simulink model "tqdtqr_rebuild_V3"  (R2021b)
settings: Solver=VariableStepAuto  StartTime=0.0  StopTime=10.0  RelTol=1e-3
undefined symbols (not defined in the file): ATQD_AfterTqMinGain_X_Deg, ATQD_APSCreepBaseTqD_X_kph, ATQD_APSCreepBaseTqD_Y_Deg, ATQD_APSCreepBaseTqR_X_kph, ATQD_APSCreepBaseTqR_Y_Deg, ATQD_APSCreepIterm_X_kph, ATQD_APSCreepIterm_Y_kph, ATQD_APSCreepPterm_X_kph, ATQD_APSCreepPterm_Y_kph, ATQD_APSDecReq_X_kph, ATQD_APSDecReq_Y_mps2, ATQD_APSDecReqCMD_X_kph, ATQD_APSDecReqTs_X_pct, ATQD_APSDecTimeGain_X_Deg, ATQD_APSDecTimeGain_Y_s, ATQD_APSReqLowSpd_X_Deg, ATQD_AutoHoldReleaseBPS_X_Deg, ATQD_AWDLoadTrqnsGain_X_kg, ATQD_AWDLoadTrqnsGain_Y_pct, ATQD_BOSEnBPSPosn_X_kph, ATQD_BOSMap_X_rpm, ATQD_BOSMap_Y_pct, ATQD_CreepBaseTqD_X_kph, ATQD_CreepBaseTqD_Y_Deg, ATQD_CreepBaseTqR_X_kph, ATQD_CreepBaseTqR_Y_Deg, ATQD_CreepBPSDisPosn_X_Deg, ATQD_CreepBPSDisPosnR_X_Deg, ATQD_CreepBPSEnPosn_X_Deg, ATQD_CreepBPSEnPosnR_X_Deg, ATQD_CreepDeltaTq_X_kph, ATQD_CreepIterm_X_kph, ATQD_CreepIterm_Y_kph, ATQD_CreepItermMaxLimit_X_pct, ATQD_CreepPreloadTime_X_kph, ATQD_CreepPreloadTq_X_kph, ATQD_CreepPreloadTq_Y_s, ATQD_CreepProtTq_X_Deg, ATQD_CreepPterm_X_kph, ATQD_CreepPterm_Y_kph, ATQD_CreepRrTqSpRat_X_rpm, ATQD_CreepRrTqSpRat_Y_Nm, ATQD_CreepTargetSpdD_X_pct, ATQD_CreepTargetSpdR_X_pct, ATQD_CreepUpLimitTq_X_rpm, ATQD_DecIneOPDHoldEnDelay_X_Deg, ATQD_DecIneOPDHoldEnDelay_Y_bar, ATQD_ECOTqMapD_X_rpm, ATQD_ECOTqMapD_Y_pct, ATQD_EMTqMapD_X_rpm, ATQD_EMTqMapD_Y_pct, ATQD_EOPDTqMapDCon_X_rpm, ATQD_EOPDTqMapDCon_Y_Deg, ATQD_EstInitVehWeight_X_c, ATQD_FAfterTqCMDGain_X_rpm, ATQD_FAfterTqCMDGain_Y_pct, ATQD_ForceLowSpd_X_Deg, ATQD_ForcePLimitSpd_X_Deg, ATQD_FrLossMAPLowV_X_rpm, ATQD_FrLossMAPLowV_Y_Nm ... (+949)
libraries: simulink x235, hcu_lib x208, tqr x63, tqd x6
(part 14 of 37)

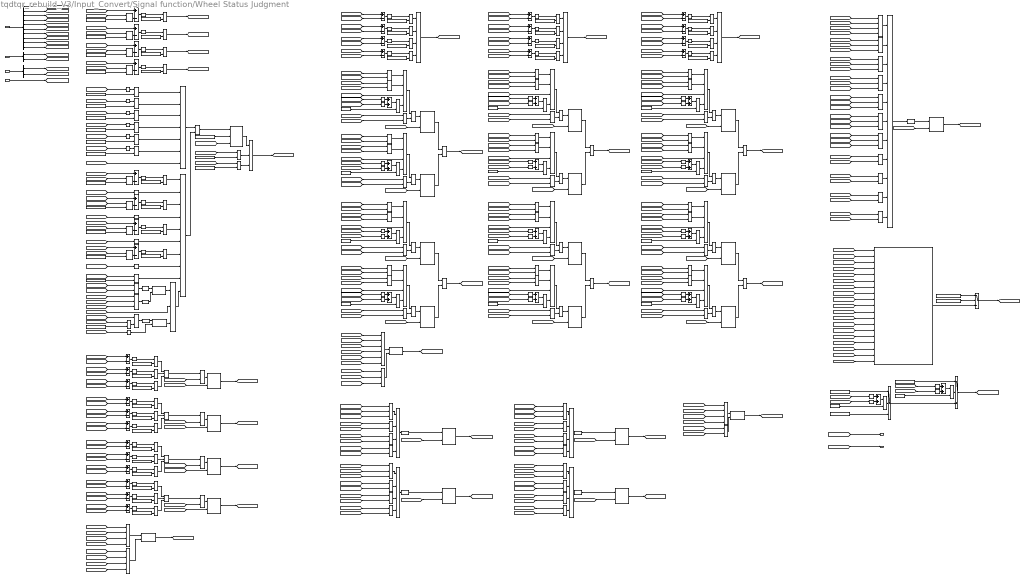
== system tqdtqr_rebuild_V3/Input_Convert/Signal function/Wheel Status Judgment ==
  note: Each wheel speed getting bigger and bigger
  note: Stable Reset Judgment
  note: Double wheels skip
  note: Skip Direction
  note: Single wheel skip
  note: Find out which wheels skip
  note: Tripple wheels skip
  note: All wheels skip
  BSCPIn_outputs : Inport
  BSignalConvert_outputs : Inport  Port=2
  BMain_outputs : Inport  Port=3
  VTQD_GearActualPosn_enum : Inport  Port=4
  AND : Logic  Inputs=7  AllPortsSameDT=off  OutDataTypeStr=boolean
  AND1 : Logic  Inputs=10  AllPortsSameDT=off  OutDataTypeStr=boolean
  AND{8,10..12,14,17,19,21,23,26,28,30,32,35..37,39..41,43..45,47..49,57..60} (29 alike) : Logic  AllPortsSameDT=off  OutDataTypeStr=boolean
  AND{6..7,9,13,15..16,18,20,22,24..25,27,29,31,33,50} (16 alike) : Logic  Inputs=4  AllPortsSameDT=off  OutDataTypeStr=boolean
  AND{2..5,34,38,42,46,51..56} (14 alike) : Logic  Inputs=3  AllPortsSameDT=off  OutDataTypeStr=boolean
  Abs{,1..37} (38 alike) : Abs
  Add{,1..23,28..31,36..39} (32 alike) : Sum  Inputs=+-
  Add{24..27,32..35,40..45} (14 alike) : Sum
  Bus Selector : BusSelector  OutputSignals=task_time_s,VINP_LFRawWhlSpeed_kph,VINP_LRRawWhlSpeed_kph,VINP_RFRawWhlSpeed_kph,VINP_RRRawWhlSpeed_kph,VINP_VehSpeed_kph,VINP_FrPTCSActive_flg,VINP_RrPTCSActive_flg,VTQD_LowIdleAccPedal_flg,VINP_DIDGetDynoMode_flg
  Bus Selector1 : BusSelector  OutputSignals=VTQD_BrkSwSta_flg,VTQD_VehActSpd_kph
  Bus Selector2 : BusSelector  OutputSignals=VTQR_NoABSFEDUWhlTqReq_Nm,VTQR_NoABSREDUWhlTqReq_Nm
  Constant{1..6,16} (7 alike) : Constant  Value=KTQD_WhlEnDetStableSpd_kph
  Constant{8,10,12,14,30,32,34,71} (8 alike) : Constant  Value=KTQD_RocModeWhlSpdDely_cnt
  Constant{9,11,13,15,17..29,38..40,46..49,54..57} (28 alike) : Constant  Value=KTQD_WhlSpeedStableDev_kph
  Constant{31,33,35..36} (4 alike) : Constant  Value=KTQD_RocModeTqLimSpdDev_kph
  Constant{41..42,44..45,50..53,58..61,64..65} (14 alike) : Constant  Value=ZERO_FLOAT
  Constant43 : Constant  Value=KTQD_FreeWhlDetStableSpd_kph
  Constant62 : Constant  Value=ENUM_GEARACTUALPOSN_N
  Constant63 : Constant  Value=ENUM_GEARACTUALPOSN_P
  Constant66 : Constant  Value=ENUM_SKIPDIRECT_NONE
  Constant67 : Constant  Value=ENUM_SKIPDIRECT_NEGATIVE
  Constant68 : Constant  Value=ENUM_SKIPDIRECT_POSITIVE
  Constant69 : Constant  Value=KTQD_ActWhlSkipSta_enum_ovrdflg
  Constant7 : Constant  Value=KTQD_WhlStableDetTime_s
  Constant70 : Constant  Value=KTQD_ActWhlSkipSta_enum_ovrdval
  Delay{,9..35} (28 alike) : Delay  DelayLength=1  InitialCondition=single(0.0)
      settings: AttributesFormatString=%<InitialCondition>
  Delay{1..8} (8 alike) : Delay  DelayLengthSource=Input port
      settings: InputPortMap=u0,p1
  DelayEnable : hcu_lib/Basic_Blocks/DelayEnable
  Detect Decrease : simulink/Logic and Bit Operations/Detect Decrease  vinit=boolean(0)  OutDataTypeStr=boolean
  Detect Increase{,1..6} (7 alike) : simulink/Logic and Bit Operations/Detect Increase  vinit=boolean(0)  OutDataTypeStr=boolean
  Equal : RelationalOperator  Operator===  OutDataTypeStr=boolean  RndMeth=Simplest
  Equal1 : RelationalOperator  Operator===  OutDataTypeStr=boolean  RndMeth=Simplest
  NOT{,1..4} (5 alike) : Logic  Operator=NOT  AllPortsSameDT=off  OutDataTypeStr=boolean
  OR{,1..4,7..10,13..21,24..29,36} (25 alike) : Logic  Operator=OR  AllPortsSameDT=off  OutDataTypeStr=boolean
  OR{11..12,23,30} (4 alike) : Logic  Operator=OR  Inputs=3  AllPortsSameDT=off  OutDataTypeStr=boolean
  OR22 : Logic  Operator=OR  Inputs=6  AllPortsSameDT=off  OutDataTypeStr=boolean
  OR{5..6,31..35} (7 alike) : Logic  Operator=OR  Inputs=4  AllPortsSameDT=off  OutDataTypeStr=boolean
  OR37 : Logic  Operator=OR  Inputs=11  AllPortsSameDT=off  OutDataTypeStr=boolean
  Relational Operator{,1..5} (6 alike) : RelationalOperator  Operator=<=  OutDataTypeStr=boolean  RndMeth=Simplest
  Relational Operator{10,31..33,38..40,48..50,54..56,64..66,70..72,77} (20 alike) : RelationalOperator  Operator=>  OutDataTypeStr=boolean  RndMeth=Simplest
  Relational Operator{11..30,37,44..47,60..63} (29 alike) : RelationalOperator  OutDataTypeStr=boolean  RndMeth=Simplest
  Relational Operator{6..9,34..36,41..43,51..53,57..59,67..69,73..76} (23 alike) : RelationalOperator  Operator=<  OutDataTypeStr=boolean  RndMeth=Simplest
  SR_Latch{,1..25} (26 alike) : hcu_lib/Basic_Blocks/SR_Latch
  Switch : Switch  Criteria=u2 ~= 0
      settings: AttributesFormatString=%<Criteria>
  Switch1 : Switch  Criteria=u2 ~= 0
      settings: AttributesFormatString=%<Criteria>
  Switch2 : Switch  Criteria=u2 ~= 0
      settings: AttributesFormatString=%<Criteria>
  Whleels State Machine : Stateflow chart  TreatAsAtomicUnit=on
  VTQD_ActWhlSkipSta_enum : Outport
  VTQD_SkipDirect_enum : Outport  Port=2
  wires:
  BSCPIn_outputs/1 -> Bus Selector/1
  Bus Selector/1 -> [task_time_s]  "<task_time_s>"
  Bus Selector/2 -> [VINP_LFRawWhlSpeed_kph]  "<VINP_LFRawWhlSpeed_kph>"
  Bus Selector/3 -> [VINP_LRRawWhlSpeed_kph]  "<VINP_LRRawWhlSpeed_kph>"
  Bus Selector/4 -> [VINP_RFRawWhlSpeed_kph]  "<VINP_RFRawWhlSpeed_kph>"
  Bus Selector/5 -> [VINP_RRRawWhlSpeed_kph]  "<VINP_RRRawWhlSpeed_kph>"
  Bus Selector/6 -> [VINP_VehSpeed_kph]  "<VINP_VehSpeed_kph>"
  Bus Selector/7 -> [VINP_FrPTCSActive_flg]  "<VINP_FrPTCSActive_flg>"
  Bus Selector/8 -> [VINP_RrPTCSActive_flg]  "<VINP_RrPTCSActive_flg>"
  Bus Selector/9 -> [VTQD_LowIdleAccPedal_flg]  "<VTQD_LowIdleAccPedal_flg>"
  BSignalConvert_outputs/1 -> Bus Selector1/1
  Bus Selector1/1 -> [VTQD_BrkSwSta_flg]  "<VTQD_BrkSwSta_flg>"
  VTQD_GearActualPosn_enum/1 -> [VTQD_GearActualPosn_enum]
  Relational Operator28/1 -> AND6/2
  Delay31/1 -> Add42/2
  [VTQD_RRWhlQuickSkip_flg] -> AND26/2
  Relational Operator20/1 -> AND3/3
  [VINP_LRRawWhlSpeed_kph] -> Relational Operator58/1
  [VINP_LFRawWhlSpeed_kph] -> Add28/1
  Constant1/1 -> Relational Operator/2
  Constant32/1 -> Delay5/2
  [VTQD_LFWhlQuickSkip_flg] -> AND17/1
  AND14/1 -> OR13/2
  [VINP_LRRawWhlSpeed_kph] -> Add22/1
  Constant40/1 -> Relational Operator30/2
  Add25/1 -> Relational Operator34/1
  NOT/1 -> AND1/2
  OR4/1 -> SR_Latch3/1
  Relational Operator40/1 -> AND13/2
  Constant28/1 -> Relational Operator24/2
  Add45/1 -> Relational Operator77/1
  Add18/1 -> Abs23/1
  Relational Operator52/1 -> AND20/1
  [VINP_VehSpeed_kph] -> Abs4/1
  Add36/1 -> Abs34/1
  Add28/1 -> Abs30/1
  [VINP_LRRawWhlSpeed_kph] -> Relational Operator33/1
  [VTQD_RRWhlQuickSkip_flg] -> AND46/3
  [VTQD_RFWhlQuickSkip_flg] -> AND19/2
  OR21/1 -> [VTQD_RearWhlSkip_flg]  "VTQD_RearWhlSkip_flg"
  OR3/1 -> SR_Latch2/1
  [VINP_LRRawWhlSpeed_kph] -> Add15/1
  [VTQD_LeftRightWhlSkip_flg] -> AND9/3
  Abs12/1 -> Relational Operator8/1
  [VTQD_RFWhlQuickSkip_flg] -> AND36/2
  AND50/1 -> OR37/1
  [VINP_LFRawWhlSpeed_kph] -> Relational Operator71/2
  [VTQD_LeftWhlSkip_flg] -> AND44/1
  AND31/1 -> OR27/1
  Abs22/1 -> Relational Operator23/1
  SR_Latch20/1 -> [VTQD_FrontLRWhlSkip_flg]  "VTQD_FrontLRWhlSkip_flg"
  Constant35/1 -> Relational Operator18/2
  Constant19/1 -> Relational Operator20/2
  Delay25/1 -> Add41/1
  [VINP_LFRawWhlSpeed_kph] -> Add20/1
  Abs36/1 -> Relational Operator62/1
  [VTQD_AllWhlStable_flg] -> OR23/3
  Constant64/1 -> Relational Operator76/2
  Constant21/1 -> Relational Operator14/2
  AND26/1 -> OR25/2
  Abs19/1 -> Relational Operator20/1
  Constant41/1 -> Relational Operator31/2
  [VTQD_LRWhlQuickSkip_flg] -> AND23/1
  Add11/1 -> Abs19/1
  Delay24/1 -> Add40/1
  [VTQD_ActWhlSkipSta_enum] -> VTQD_ActWhlSkipSta_enum/1
  [VINP_LRRawWhlSpeed_kph] -> Add1/1
  Abs32/1 -> Relational Operator46/1
  [VTQD_AllWhlStable_flg] -> SR_Latch1/2
  [VINP_LRRawWhlSpeed_kph] -> Add9/2
  [VTQD_LeftWhlSkip_flg] -> OR22/1
  AND23/1 -> OR19/2
  Abs/1 -> Relational Operator/1
  [VTQD_RFWhlQuickSkip_flg] -> AND30/1
  [VINP_RFRawWhlSpeed_kph] -> Add13/1
  [VINP_LFRawWhlSpeed_kph] -> Add10/1
  NOT3/1 -> AND1/8
  Add33/1 -> Relational Operator51/1
  [VINP_RRRawWhlSpeed_kph] -> Add29/2
  [VTQD_RightWhlSkip_flg] -> OR22/2
  Constant5/1 -> Relational Operator4/2
  [VINP_RRRawWhlSpeed_kph] -> Add11/2
  [VINP_LFRawWhlSpeed_kph] -> Add8/1
  Add22/1 -> Abs28/1
  Constant38/1 -> Relational Operator28/2
  [VINP_RFRawWhlSpeed_kph] -> Add30/1
  Abs15/1 -> Relational Operator12/1
  [VTQD_TripleWhlSkip_flg] -> OR23/1
  Relational Operator21/1 -> AND4/1
  AND18/1 -> OR16/1
  Equal/1 -> OR30/2
  [VINP_RFRawWhlSpeed_kph] -> Add19/2
  SR_Latch22/1 -> [VTQD_RearLFWhlSkip_flg]  "VTQD_RearLFWhlSkip_flg"
  [VTQD_LRWhlQuickSkip_flg] -> AND45/2
  OR10/1 -> Detect Decrease/1
  [VTQD_RFLRWhlSkip_flg] -> AND56/1
  Constant8/1 -> Delay2/2
  Relational Operator9/1 -> AND1/7
  AND/1 -> OR/1
  AND3/1 -> OR2/1
  Abs6/1 -> Relational Operator16/1
  AND4/1 -> OR3/1
  Delay7/1 -> Add6/2
  Relational Operator51/1 -> AND20/4
  [VTQD_LeftWhlSkip_flg] -> AND36/1
  [VTQD_LRWhlQuickSkip_flg] -> OR3/2
  [VINP_VehSpeed_kph] -> Delay7/1
  OR19/1 -> SR_Latch13/1
  Add6/1 -> Abs12/1
  AND34/1 -> OR31/1
  AND11/1 -> Detect Increase1/1
  Abs21/1 -> Relational Operator22/1
  AND48/1 -> OR34/3
  Relational Operator16/1 -> [VTQD_LRWhlQuickSkip_flg]  "VTQD_LRWhlQuickSkip_flg"
  [VINP_RRRawWhlSpeed_kph] -> Abs3/1
  [VTQD_RRWhlQuickSkip_flg] -> AND12/2
  Relational Operator35/1 -> AND9/1
  Add35/1 -> Relational Operator57/1
  [VTQD_FrontWhlSkip_flg] -> AND39/1
  [VTQD_LFWhlQuickSkip_flg] -> AND8/1
  Add4/1 -> Abs10/1
  [VINP_RFRawWhlSpeed_kph] -> Add31/1
  Constant69/1 -> Switch2/2
  Abs33/1 -> Relational Operator47/1
  [VTQR_NoABSFEDUWhlTqReq_Nm] -> Delay10/1
  Delay14/1 -> Add27/2
  [VINP_LRRawWhlSpeed_kph] -> Delay4/1
  [VTQD_LRWhlQuickSkip_flg] -> AND55/3
  [VTQD_LRWhlQuickSkip_flg] -> AND34/3
  AND51/1 -> OR37/2
  AND32/1 -> OR27/2
  Delay11/1 -> Add25/2
  [VTQD_DiagonalWhlSkip_flg] -> AND29/3
  [VTQD_LeftWhlSkip_flg] -> Whleels State Machine/6(VTQD_LeftWhlSkip_flg)
  [VINP_LFRawWhlSpeed_kph] -> Relational Operator65/1
  Relational Operator23/1 -> AND4/3
  Delay13/1 -> Add27/1
  [VTQD_LowIdleAccPedal_flg] -> AND11/1
  [VTQD_LRWhlQuickSkip_flg] -> AND52/3
  [VTQD_AllWhlStable_flg] -> SR_Latch21/2
  [VINP_RRRawWhlSpeed_kph] -> Relational Operator56/1
  AND40/1 -> OR32/3
  Relational Operator15/1 -> [VTQD_LFWhlQuickSkip_flg]  "VTQD_LFWhlQuickSkip_flg"
  Relational Operator47/1 -> AND16/4
  Relational Operator11/1 -> AND2/1
  Add34/1 -> Relational Operator54/1
  Constant46/1 -> Relational Operator44/2
  Constant15/1 -> Relational Operator9/2
  Abs28/1 -> Relational Operator29/1
  [VTQD_RFWhlQuickSkip_flg] -> AND51/2
  [VTQD_RRWhlQuickSkip_flg] -> AND44/2
  [VINP_RFRawWhlSpeed_kph] -> Relational Operator50/1
  [VINP_RFRawWhlSpeed_kph] -> Relational Operator42/1
  [VINP_RFRawWhlSpeed_kph] -> Add36/2
  [VTQD_FrontLRWhlSkip_flg] -> AND57/1
  Detect Increase4/1 -> SR_Latch22/1
  Relational Operator45/1 -> AND16/2
  OR12/1 -> AND1/10
  Delay30/1 -> Add43/2
  [VTQD_LFWhlQuickSkip_flg] -> AND43/2
  [VINP_LFRawWhlSpeed_kph] -> Relational Operator39/2
  [VTQD_RRWhlQuickSkip_flg] -> AND42/3
  Constant39/1 -> Relational Operator29/2
  [VTQD_RRWhlSkip_flg] -> OR5/4
  OR27/1 -> SR_Latch18/1
  Delay35/1 -> Add45/2
  [VTQD_RRWhlQuickSkip_flg] -> AND50/4
  Relational Operator8/1 -> AND1/5
  [VTQD_RightWhlSkip_flg] -> AND48/1
  [VTQD_LeftRightWhlSkip_flg] -> AND13/3
  AND57/1 -> OR37/8
  Relational Operator4/1 -> AND/5
  [VTQD_RearLFWhlSkip_flg] -> OR35/3
  Add2/1 -> Abs7/1
  [VTQD_VehActSpd_kph] -> Abs9/1
  [VTQD_RFWhlQuickSkip_flg] -> AND34/2
  [VTQD_LFRRWhlSkip_flg] -> OR22/5
  AND15/1 -> OR14/1
  Relational Operator36/1 -> AND9/2
  Constant27/1 -> Relational Operator26/2
  Add14/1 -> Abs22/1
  [VINP_RRRawWhlSpeed_kph] -> Relational Operator36/2
  Relational Operator76/1 -> Switch/2
  [VTQD_RearWhlSkip_flg] -> OR22/4
  [VTQD_AllWhlStable_flg] -> SR_Latch17/2
  NOT1/1 -> AND1/4
  Constant68/1 -> Switch1/1
  [VTQD_LFWhlQuickSkip_flg] -> OR1/2
  Detect Increase/1 -> SR_Latch7/2
  Constant14/1 -> Delay3/2
  Relational Operator19/1 -> AND3/2
  OR2/1 -> SR_Latch1/1
  SR_Latch13/1 -> OR21/1  "VTQD_PosRearWhlSkip_flg"
  [VTQD_VehActSpd_kph] -> Relational Operator10/1
  [VTQD_RFWhlQuickSkip_flg] -> AND17/2
  [VTQR_NoABSREDUWhlTqReq_Nm] -> Delay26/1
  AND8/1 -> OR7/2
  Constant50/1 -> Relational Operator48/2
  Delay2/1 -> Add5/2
  [VTQD_RFWhlQuickSkip_flg] -> AND55/2
  [VTQD_LFRRWhlSkip_flg] -> AND45/1
  OR22/1 -> SR_Latch15/1
  Relational Operator34/1 -> AND9/4
  Constant56/1 -> Relational Operator62/2
  Constant54/1 -> Relational Operator60/2
  Relational Operator77/1 -> Switch1/2
  NOT4/1 -> SR_Latch8/2
  AND30/1 -> OR28/2
  Add29/1 -> Abs31/1
  Abs16/1 -> Relational Operator13/1
  [VTQD_AllWhlStable_flg] -> SR_Latch12/2
  AND33/1 -> OR28/1
  [VTQR_NoABSFEDUWhlTqReq_Nm] -> Delay28/1
  AND16/1 -> [VTQD_FrontRearWhlSkip_flg]  "VTQD_FrontRearWhlSkip_flg"
  Delay34/1 -> Add45/1
  Relational Operator68/1 -> AND29/1
  [VINP_RrPTCSActive_flg] -> OR10/2
  Abs13/1 -> Relational Operator9/1
  [VINP_RFRawWhlSpeed_kph] -> Relational Operator74/1
  Delay32/1 -> Add44/1
  [VTQD_SingleWhlSkip_flg] -> Whleels State Machine/5(VTQD_SingleWhlSkip_flg)
  [VINP_RRRawWhlSpeed_kph] -> Relational Operator72/2
  Relational Operator65/1 -> AND27/1
  [VTQR_NoABSREDUWhlTqReq_Nm] -> Delay17/1
  [VINP_LRRawWhlSpeed_kph] -> Relational Operator52/2
  Add5/1 -> Abs11/1
  Delay17/1 -> Add33/2
  [VINP_RRRawWhlSpeed_kph] -> Relational Operator66/1
  [VINP_LRRawWhlSpeed_kph] -> Add17/2
  Add9/1 -> Abs15/1
  AND60/1 -> OR37/11
  AND29/1 -> OR25/1
  [VTQD_AllWhlStable_flg] -> SR_Latch2/2
  [VTQR_NoABSFEDUWhlTqReq_Nm] -> Delay/1
  [VTQD_LeftWhlSkip_flg] -> AND51/1
  Add/1 -> Abs5/1
  [VINP_RFRawWhlSpeed_kph] -> Add22/2
  Relational Operator59/1 -> AND24/2
  SR_Latch1/1 -> [VTQD_RFWhlSkip_flg]  "VTQD_RFWhlSkip_flg"
  Constant44/1 -> Relational Operator38/2
  Add41/1 -> Relational Operator67/1
  Constant9/1 -> Relational Operator6/2
  Constant10/1 -> Delay7/2
  Abs2/1 -> Relational Operator2/1
  Constant49/1 -> Relational Operator47/2
  [VTQD_RearRFWhlSkip_flg] -> AND60/1
  [VINP_RRRawWhlSpeed_kph] -> Add14/2
  Relational Operator29/1 -> AND6/3
  SR_Latch15/1 -> [VTQD_DoubleWhlSkip_flg]  "VTQD_DoubleWhlSkip_flg"
  [VINP_LFRawWhlSpeed_kph] -> Relational Operator68/1
  Detect Increase5/1 -> SR_Latch23/1
  [VINP_RFRawWhlSpeed_kph] -> Relational Operator53/1
  [VTQD_AllWhlStable_flg] -> SR_Latch14/2
  [VTQR_NoABSFEDUWhlTqReq_Nm] -> Delay18/1
  [VTQD_AllWhlStable_flg] -> SR_Latch13/2
  [VTQD_FrontWhlSkip_flg] -> AND53/1
  AND52/1 -> OR37/3
  Relational Operator33/1 -> AND7/2
  Constant31/1 -> Relational Operator15/2
  [VTQD_RearRFWhlSkip_flg] -> Whleels State Machine/16(VTQD_RearRFWhlSkip_flg)
  Add19/1 -> Abs24/1
  [VTQD_LeftRightWhlSkip_flg] -> AND7/3
  DelayEnable/1 -> OR30/1
  [VINP_RFRawWhlSpeed_kph] -> Relational Operator39/1
  Relational Operator2/1 -> AND/3
  [VINP_LRRawWhlSpeed_kph] -> Add30/2
  [VTQR_NoABSREDUWhlTqReq_Nm] -> Delay31/1
  Constant48/1 -> Relational Operator46/2
  [VINP_RFRawWhlSpeed_kph] -> Relational Operator32/2
  [VTQD_FrontRRWhlSkip_flg] -> Whleels State Machine/14(VTQD_FrontRRWhlSkip_flg)
  [VTQD_LFWhlQuickSkip_flg] -> AND19/1
  Constant58/1 -> Relational Operator64/2
  [VINP_RFRawWhlSpeed_kph] -> Delay5/1
  [VTQD_FrontWhlSkip_flg] -> Whleels State Machine/8(VTQD_FrontWhlSkip_flg)
  Delay6/1 -> Add3/2
  [VTQD_DoubleWhlSkip_flg] -> Whleels State Machine/12(VTQD_DoubleWhlSkip_flg)
  [VINP_RRRawWhlSpeed_kph] -> Relational Operator43/1
  [VTQD_RFWhlQuickSkip_flg] -> AND41/2
  [VINP_LRRawWhlSpeed_kph] -> Add13/2
  [VINP_FrPTCSActive_flg] -> OR10/1
  [VTQD_FrontLRWhlSkip_flg] -> OR35/1
  [VINP_RRRawWhlSpeed_kph] -> Relational Operator50/2
  OR9/1 -> [VTQD_LeftWhlSkip_flg]  "VTQD_LeftWhlSkip_flg"
  AND39/1 -> OR32/2
  Constant29/1 -> Relational Operator27/2
  Relational Operator50/1 -> AND18/2
  SR_Latch5/1 -> OR9/1  "VTQD_PosLeftWhlSkip_flg"
  [VTQD_RFLRWhlSkip_flg] -> AND37/1
  [VTQD_AllWhlStable_flg] -> SR_Latch3/2
  Relational Operator31/1 -> AND7/4
  [VTQD_LRWhlQuickSkip_flg] -> AND32/2
  [VTQD_RFWhlQuickSkip_flg] -> AND32/1
  [VINP_RFRawWhlSpeed_kph] -> Relational Operator71/1
  [VTQD_RRWhlQuickSkip_flg] -> AND39/2
  [VINP_LFRawWhlSpeed_kph] -> Add/1
  OR18/1 -> [VTQD_FrontWhlSkip_flg]  "VTQD_FrontWhlSkip_flg"
  AND47/1 -> OR34/2
  [VTQD_RearWhlSkip_flg] -> AND54/1
  Constant26/1 -> Relational Operator25/2
  SR_Latch18/1 -> OR29/1  "VTQD_PosRFLRWhlSkip_flg"
  [VINP_RFRawWhlSpeed_kph] -> Abs1/1
  OR17/1 -> SR_Latch12/1
  Relational Operator72/1 -> AND31/2
  Relational Operator3/1 -> AND/4
  Delay5/1 -> Add2/2
  [VTQD_DiagonalWhlSkip_flg] -> AND27/3
  [VINP_LFRawWhlSpeed_kph] -> Add37/1
  [VTQD_RRWhlQuickSkip_flg] -> AND21/2
  [VINP_RRRawWhlSpeed_kph] -> Relational Operator75/2
  Add10/1 -> Abs16/1
  [VTQD_LFWhlQuickSkip_flg] -> AND56/2
  Constant36/1 -> Relational Operator16/2
  Switch1/1 -> [VTQD_SkipDirect_enum]  "VTQD_SkipDirect_enum"
  Delay20/1 -> Add34/1
  [VTQD_DiagonalWhlSkip_flg] -> AND33/3
  [VTQR_NoABSREDUWhlTqReq_Nm] -> Delay15/1
  [VINP_RFRawWhlSpeed_kph] -> Relational Operator56/2
  Relational Operator70/1 -> AND31/4
  SR_Latch16/1 -> OR26/1  "VTQD_PosLFRRWhlSkip_flg"
  SR_Latch25/1 -> [VTQD_AllWhlSkip_flg]  "VTQD_AllWhlSkip_flg"
  [VINP_LRRawWhlSpeed_kph] -> Relational Operator49/2
  [VTQD_RFWhlSkip_flg] -> Whleels State Machine/2(VTQD_RFWhlSkip_flg)
  Constant70/1 -> Switch2/1
  [VTQD_AllWhlStable_flg] -> SR_Latch/2
  Relational Operator13/1 -> AND2/3
  Delay27/1 -> Add40/2
  Add17/1 -> Abs25/1
  [VTQD_FrontRearWhlSkip_flg] -> AND20/3
  AND2/1 -> OR1/1
  [VINP_RRRawWhlSpeed_kph] -> Add23/2
  [VTQR_NoABSFEDUWhlTqReq_Nm] -> Delay29/1
  Delay28/1 -> Add42/1
  [VTQD_FrontWhlSkip_flg] -> AND35/1
  [VTQD_AllWhlStable_flg] -> SR_Latch22/2
  Add39/1 -> Abs37/1
  Constant52/1 -> Relational Operator54/2
  [VTQD_AllWhlStable_flg] -> SR_Latch25/2
  [VTQD_RFWhlSkip_flg] -> OR5/2
  AND49/1 -> OR34/4
  [VINP_RRRawWhlSpeed_kph] -> Add19/1
  [VTQD_FrontRRWhlSkip_flg] -> OR35/2
  [VTQD_RearWhlSkip_flg] -> Whleels State Machine/9(VTQD_RearWhlSkip_flg)
  Constant17/1 -> Relational Operator19/2
  [VTQD_LFWhlQuickSkip_flg] -> AND34/1
  Delay18/1 -> Add33/1
  [VTQD_RearLFWhlSkip_flg] -> Whleels State Machine/15(VTQD_RearLFWhlSkip_flg)
  [VTQD_AllWhlSkip_flg] -> OR6/3
  Add43/1 -> Relational Operator73/1
  [VTQD_RFWhlQuickSkip_flg] -> AND50/2
  [VTQD_RFWhlQuickSkip_flg] -> AND12/1
  Relational Operator38/1 -> AND13/4
  OR25/1 -> SR_Latch17/1
  [VTQD_RFWhlQuickSkip_flg] -> AND54/3
  Switch2/1 -> [VTQD_ActWhlSkipSta_enum]  "VTQD_ActWhlSkipSta_enum"
  Add16/1 -> Abs21/1
  [VTQD_RRWhlQuickSkip_flg] -> AND23/2
  Constant42/1 -> Relational Operator34/2
  [VTQD_AllWhlStable_flg] -> SR_Latch5/2
  [VINP_RRRawWhlSpeed_kph] -> Add10/2
  [VINP_RrPTCSActive_flg] -> OR11/2
  AND42/1 -> OR33/1
  [VTQD_AllWhlStable_flg] -> SR_Latch23/2
  Delay16/1 -> Add32/1
  SR_Latch23/1 -> [VTQD_RearRFWhlSkip_flg]  "VTQD_RearRFWhlSkip_flg"
  Abs30/1 -> Relational Operator44/1
  AND54/1 -> OR37/5
  [VTQD_RFWhlQuickSkip_flg] -> AND47/2
  Constant45/1 -> Relational Operator41/2
  AND20/1 -> OR17/1
  AND17/1 -> OR17/2
  Relational Operator49/1 -> AND18/1
  Constant51/1 -> Relational Operator51/2
  [VTQD_RRWhlQuickSkip_flg] -> OR4/2
  [VTQD_LFWhlQuickSkip_flg] -> AND26/1
  OR14/1 -> SR_Latch10/1
  Relational Operator69/1 -> AND29/2
  Constant60/1 -> Relational Operator70/2
  [VINP_LFRawWhlSpeed_kph] -> Relational Operator42/2
  Relational Operator26/1 -> AND5/3
  Delay/1 -> Add24/1
  AND55/1 -> OR37/6
  [VTQD_AllWhlStable_flg] -> OR36/2
  Add3/1 -> Abs8/1
  [VTQD_RFLRWhlSkip_flg] -> AND49/1
  SR_Latch3/1 -> [VTQD_RRWhlSkip_flg]  "VTQD_RRWhlSkip_flg"
  [VINP_RFRawWhlSpeed_kph] -> Add8/2
  [VINP_RRRawWhlSpeed_kph] -> Relational Operator59/1
  [VINP_RFRawWhlSpeed_kph] -> Add5/1
  [VINP_LRRawWhlSpeed_kph] -> Relational Operator69/2
  Constant65/1 -> Relational Operator77/2
  SR_Latch21/1 -> [VTQD_FrontRRWhlSkip_flg]  "VTQD_FrontRRWhlSkip_flg"
  [VTQR_NoABSFEDUWhlTqReq_Nm] -> Delay13/1
  OR37/1 -> Detect Increase6/1
  [VINP_RRRawWhlSpeed_kph] -> Add3/1
  [VTQD_AllWhlStable_flg] -> SR_Latch6/2
  OR/1 -> DelayEnable/1
  OR24/1 -> SR_Latch16/1
  [VTQD_RRWhlQuickSkip_flg] -> AND57/2
  Add12/1 -> Abs17/1
  [VTQD_FrontRearWhlSkip_flg] -> AND24/3
  [VTQD_RearWhlSkip_flg] -> AND43/1
  Add21/1 -> Abs27/1
  [VTQD_SkipDirect_enum] -> VTQD_SkipDirect_enum/1
  OR28/1 -> SR_Latch19/1
  Constant7/1 -> DelayEnable/2
  [VTQD_FrontRearWhlSkip_flg] -> AND22/3
  [VINP_LRRawWhlSpeed_kph] -> Relational Operator55/1
  [VINP_RFRawWhlSpeed_kph] -> Relational Operator68/2
  [VTQD_RearWhlSkip_flg] -> AND47/1
  [VINP_RFRawWhlSpeed_kph] -> Add16/2
  [VINP_RRRawWhlSpeed_kph] -> Add39/1
  Delay21/1 -> Add35/1
  [VTQD_LFWhlQuickSkip_flg] -> NOT/1
  [VINP_LFRawWhlSpeed_kph] -> Add18/2
  AND43/1 -> OR33/2
  Relational Operator24/1 -> AND5/1
  [VTQD_LFWhlQuickSkip_flg] -> AND52/2
  Equal1/1 -> OR30/3
  [VTQD_RFWhlQuickSkip_flg] -> AND59/2
  Relational Operator39/1 -> AND13/1
  Relational Operator7/1 -> AND1/3
  AND5/1 -> OR4/1
  Constant16/1 -> Relational Operator10/2
  Delay9/1 -> Add24/2
  [VTQD_LRWhlQuickSkip_flg] -> AND46/2
  AND53/1 -> OR37/4
  Add13/1 -> Abs18/1
  Relational Operator75/1 -> AND33/2
  SR_Latch9/1 -> OR15/1  "VTQD_PosRightWhlSkip_flg"
  Relational Operator53/1 -> AND20/2
  [VTQD_TripleWhlSkip_flg] -> OR6/2
  Detect Increase3/1 -> SR_Latch21/1
  Add37/1 -> Abs35/1
  [VTQR_NoABSREDUWhlTqReq_Nm] -> Delay19/1
  [VINP_LRRawWhlSpeed_kph] -> Relational Operator72/1
  [VTQD_AllWhlStable_flg] -> SR_Latch19/2
  OR16/1 -> SR_Latch11/1
  [VTQD_RFWhlQuickSkip_flg] -> OR2/2
  [VINP_LFRawWhlSpeed_kph] -> Add36/1
  OR13/1 -> SR_Latch9/1
  Relational Operator10/1 -> AND1/9
  Constant67/1 -> Switch/1
  OR8/1 -> SR_Latch6/1
  [VINP_RFRawWhlSpeed_kph] -> Add11/1
  [VTQD_AllWhlStable_flg] -> SR_Latch20/2
  [VTQR_NoABSFEDUWhlTqReq_Nm] -> Delay25/1
  Add8/1 -> Abs14/1
  Add26/1 -> Relational Operator38/1
  Add1/1 -> Abs6/1
  Add38/1 -> Abs36/1
  Constant13/1 -> Relational Operator8/2
  [VTQD_RRWhlQuickSkip_flg] -> AND28/2
  Relational Operator63/1 -> AND25/4
  AND41/1 -> OR32/4
  [VINP_VehSpeed_kph] -> Delay2/1
  SR_Latch12/1 -> OR18/2  "VTQD_NegFrontWhlSkip_flg"
  [VTQD_AllWhlStable_flg] -> SR_Latch10/2
  [VINP_LFRawWhlSpeed_kph] -> Relational Operator58/2
  Delay10/1 -> Add25/1
  SR_Latch4/1 -> [VTQD_SingleWhlSkip_flg]  "VTQD_SingleWhlSkip_flg"
  [VTQD_TripleWhlSkip_flg] -> Whleels State Machine/17(VTQD_TripleWhlSkip_flg)
  [task_time_s] -> DelayEnable/3
  AND22/1 -> OR19/1
  [VINP_VehSpeed_kph] -> Delay1/1
  [VINP_LFRawWhlSpeed_kph] -> Add12/2
  [VINP_LFRawWhlSpeed_kph] -> Add21/1
  [VINP_LFRawWhlSpeed_kph] -> Add29/1
  Add23/1 -> Abs29/1
  [VTQD_RFWhlQuickSkip_flg] -> AND38/2
  Constant33/1 -> Relational Operator17/2
  [VTQD_LRWhlQuickSkip_flg] -> AND35/2
  [VINP_LRRawWhlSpeed_kph] -> Add28/2
  Relational Operator54/1 -> AND22/4
  Delay29/1 -> Add43/1
  Relational Operator73/1 -> AND33/4
  Relational Operator61/1 -> AND25/2
  [VTQR_NoABSREDUWhlTqReq_Nm] -> Delay14/1
  [VTQD_DiagonalWhlSkip_flg] -> AND31/3
  AND27/1 -> OR24/1
  OR5/1 -> SR_Latch4/1
  [VINP_LRRawWhlSpeed_kph] -> Relational Operator36/1
  AND37/1 -> OR31/4
  Relational Operator25/1 -> AND5/2
  [VTQR_NoABSFEDUWhlTqReq_Nm] -> Delay16/1
  Abs14/1 -> Relational Operator11/1
  Abs24/1 -> Relational Operator25/1
  [VINP_RFRawWhlSpeed_kph] -> Add2/1
  OR20/1 -> SR_Latch14/1
  SR_Latch17/1 -> OR26/2  "VTQD_NegLFRRWhlSkip_flg"
  Relational Operator66/1 -> AND27/2
  [VTQD_FrontRRWhlSkip_flg] -> AND58/1
  Relational Operator48/1 -> AND18/4
  [VTQD_RFLRWhlSkip_flg] -> Whleels State Machine/11(VTQD_RFLRWhlSkip_flg)
  AND21/1 -> OR20/2
  [VINP_RRRawWhlSpeed_kph] -> Add7/1
  [VINP_LFRawWhlSpeed_kph] -> Add4/1
  Detect Increase1/1 -> SR_Latch8/1
  Constant62/1 -> Equal/2
  [VTQR_NoABSREDUWhlTqReq_Nm] -> Delay30/1
  Constant59/1 -> Relational Operator67/2
  Abs4/1 -> Relational Operator4/1
  Switch/1 -> Switch1/3
  OR34/1 -> Detect Increase5/1
  Abs1/1 -> Relational Operator1/1
  [VTQD_RRWhlQuickSkip_flg] -> AND51/3
  [VINP_RFRawWhlSpeed_kph] -> Relational Operator35/2
  SR_Latch/1 -> [VTQD_LFWhlSkip_flg]  "VTQD_LFWhlSkip_flg"
  Abs27/1 -> Relational Operator28/1
  [VTQD_LowIdleAccPedal_flg] -> NOT4/1
  [VTQD_LFWhlQuickSkip_flg] -> AND40/2
  [VINP_RRRawWhlSpeed_kph] -> Relational Operator69/1
  [VTQD_AllWhlStable_flg] -> SR_Latch18/2
  Constant4/1 -> Relational Operator3/2
  Constant22/1 -> Relational Operator11/2
  [VTQD_AllWhlStable_flg] -> OR6/4
  [VTQD_LeftRightWhlSkip_flg] -> AND15/3
  [VINP_LFRawWhlSpeed_kph] -> Relational Operator35/1
  [VTQD_LRWhlQuickSkip_flg] -> NOT1/1
  [VINP_LFRawWhlSpeed_kph] -> Delay3/1
  [VTQD_BrkSwSta_flg] -> OR12/2
  [VINP_LFRawWhlSpeed_kph] -> Add9/1
  Constant57/1 -> Relational Operator63/2
  OR6/1 -> SR_Latch4/2
  Constant66/1 -> Switch/3
  Constant2/1 -> Relational Operator1/2
  [VTQD_LFWhlSkip_flg] -> OR5/1
  [VTQD_AllWhlSkip_flg] -> OR23/2
  [VTQR_NoABSREDUWhlTqReq_Nm] -> Delay9/1
  Relational Operator/1 -> AND/1
  [VTQR_NoABSFEDUWhlTqReq_Nm] -> Delay32/1
  [VTQD_FrontWhlSkip_flg] -> OR22/3
  [VTQD_LRWhlQuickSkip_flg] -> AND42/2
  [VINP_LRRawWhlSpeed_kph] -> Relational Operator75/1
  [VINP_LRRawWhlSpeed_kph] -> Add39/2
  Relational Operator18/1 -> [VTQD_RRWhlQuickSkip_flg]  "VTQD_RRWhlQuickSkip_flg"
  [VTQD_RightWhlSkip_flg] -> Whleels State Machine/7(VTQD_RightWhlSkip_flg)
  [VINP_RRRawWhlSpeed_kph] -> Add38/1
  [VTQD_LRWhlQuickSkip_flg] -> AND30/2
  [VTQD_LRWhlQuickSkip_flg] -> AND8/2
  [VTQR_NoABSREDUWhlTqReq_Nm] -> Delay23/1
  [VINP_LFRawWhlSpeed_kph] -> Relational Operator49/1
  Relational Operator57/1 -> AND24/4
  OR11/1 -> Detect Increase/1
  Abs26/1 -> Relational Operator27/1
  [VTQD_LRWhlQuickSkip_flg] -> AND21/1
  [VTQD_VehActSpd_kph] -> Relational Operator37/1
  Abs25/1 -> Relational Operator26/1
  Relational Operator62/1 -> AND25/3
  Abs18/1 -> Relational Operator19/1
  Constant11/1 -> Relational Operator7/2
  SR_Latch14/1 -> OR21/2  "VTQD_NegRearWhlSkip_flg"
  Abs29/1 -> Relational Operator30/1
  AND1/1 -> OR/2
  OR1/1 -> SR_Latch/1
  [VINP_LFRawWhlSpeed_kph] -> Relational Operator55/2
  Add30/1 -> Abs32/1
  [VTQR_NoABSREDUWhlTqReq_Nm] -> Delay35/1
  [VINP_LFRawWhlSpeed_kph] -> Abs/1
  Constant47/1 -> Relational Operator45/2
  Constant53/1 -> Relational Operator57/2
  Relational Operator58/1 -> AND24/1
  [VTQD_AllWhlSkip_flg] -> Whleels State Machine/18(VTQD_AllWhlSkip_flg)
  AND38/1 -> OR32/1
  Add15/1 -> Abs20/1
  [VTQR_NoABSREDUWhlTqReq_Nm] -> Delay22/1
  Add27/1 -> Relational Operator41/1
  [VTQD_RRWhlQuickSkip_flg] -> AND56/3
  Relational Operator5/1 -> AND/6
  AND45/1 -> OR33/4
  Delay4/1 -> Add1/2
  Abs23/1 -> Relational Operator24/1
  Abs11/1 -> Relational Operator7/1
  AND13/1 -> OR13/1
  Add7/1 -> Abs13/1
  [VINP_LFRawWhlSpeed_kph] -> Relational Operator74/2
  [VTQD_RightWhlSkip_flg] -> AND52/1
  [VINP_RRRawWhlSpeed_kph] -> Add18/1
  AND19/1 -> OR16/2
  AND6/1 -> [VTQD_LeftRightWhlSkip_flg]  "VTQD_LeftRightWhlSkip_flg"
  Abs31/1 -> Relational Operator45/1
  [VTQD_AllWhlStable_flg] -> SR_Latch16/2
  AND58/1 -> OR37/9
  AND44/1 -> OR33/3
  [VINP_RFRawWhlSpeed_kph] -> Add38/2
  Relational Operator64/1 -> AND27/4
  [VINP_RFRawWhlSpeed_kph] -> Add20/2
  Delay15/1 -> Add26/2
  Relational Operator55/1 -> AND22/1
  AND46/1 -> OR34/1
  [VTQD_RFWhlQuickSkip_flg] -> NOT2/1
  [VTQD_LFWhlQuickSkip_flg] -> AND50/1
  OR26/1 -> [VTQD_LFRRWhlSkip_flg]  "VTQD_LFRRWhlSkip_flg"
  SR_Latch7/1 -> OR12/1
  [VTQD_GearActualPosn_enum] -> Equal/1
  Relational Operator44/1 -> AND16/1
  [VINP_LRRawWhlSpeed_kph] -> Add37/2
  Abs5/1 -> Relational Operator15/1
  [VTQD_LRWhlSkip_flg] -> Whleels State Machine/3(VTQD_LRWhlSkip_flg)
  [VTQD_LFRRWhlSkip_flg] -> Whleels State Machine/10(VTQD_LFRRWhlSkip_flg)
  Relational Operator27/1 -> AND6/1
  [VTQD_RRWhlQuickSkip_flg] -> AND38/3
  [VTQD_RRWhlQuickSkip_flg] -> AND14/2
  [VINP_LRRawWhlSpeed_kph] -> Relational Operator43/2
  SR_Latch2/1 -> [VTQD_LRWhlSkip_flg]  "VTQD_LRWhlSkip_flg"
  Relational Operator17/1 -> [VTQD_RFWhlQuickSkip_flg]  "VTQD_RFWhlQuickSkip_flg"
  Add42/1 -> Relational Operator70/1
  Abs37/1 -> Relational Operator63/1
  Constant20/1 -> Relational Operator13/2
  [VTQD_LRWhlQuickSkip_flg] -> AND58/2
  Constant23/1 -> Relational Operator22/2
  AND59/1 -> OR37/10
  Constant34/1 -> Delay6/2
  Relational Operator60/1 -> AND25/1
  [VTQD_BrkSwSta_flg] -> AND/7
  [VTQD_LFWhlSkip_flg] -> Whleels State Machine/1(VTQD_LFWhlSkip_flg)
  AND9/1 -> OR8/1
  Delay12/1 -> Add26/1
  Add20/1 -> Abs26/1
  Relational Operator74/1 -> AND33/1
  [VTQD_RRWhlQuickSkip_flg] -> AND49/2
  AND36/1 -> OR31/3
  [VINP_LRRawWhlSpeed_kph] -> Relational Operator40/2
  [VTQD_LFWhlQuickSkip_flg] -> AND38/1
  Relational Operator12/1 -> AND2/2
  Constant30/1 -> Delay4/2
  Abs9/1 -> Relational Operator5/1
  [VTQD_AllWhlStable_flg] -> SR_Latch9/2
  [VINP_RRRawWhlSpeed_kph] -> Relational Operator40/1
  [VTQR_NoABSFEDUWhlTqReq_Nm] -> Delay24/1
  [VINP_RRRawWhlSpeed_kph] -> Relational Operator33/2
  AND56/1 -> OR37/7
  [VINP_LRRawWhlSpeed_kph] -> Abs2/1
  Add24/1 -> Relational Operator31/1
  [VTQR_NoABSFEDUWhlTqReq_Nm] -> Delay21/1
  Relational Operator1/1 -> AND/2
  Add32/1 -> Relational Operator48/1
  [VTQD_LRWhlSkip_flg] -> OR5/3
  Delay8/1 -> Add7/2
  [VTQD_LRWhlQuickSkip_flg] -> AND48/2
  [VTQD_RRWhlSkip_flg] -> Whleels State Machine/4(VTQD_RRWhlSkip_flg)
  [VTQD_LFWhlQuickSkip_flg] -> AND28/1
  [VTQD_FrontLRWhlSkip_flg] -> Whleels State Machine/13(VTQD_FrontLRWhlSkip_flg)
  [VTQD_AllWhlStable_flg] -> SR_Latch11/2
  Abs7/1 -> Relational Operator17/1
  Abs8/1 -> Relational Operator18/1
  [VTQD_RFWhlQuickSkip_flg] -> AND46/1
  OR7/1 -> SR_Latch5/1
  [VTQD_LFRRWhlSkip_flg] -> AND55/1
  NOT2/1 -> AND1/6
  [VINP_RFRawWhlSpeed_kph] -> Relational Operator59/2
  OR31/1 -> Detect Increase2/1
  Relational Operator43/1 -> AND15/2
  Add44/1 -> Relational Operator76/1
  [VTQD_LRWhlQuickSkip_flg] -> AND53/2
  Abs3/1 -> Relational Operator3/1
  OR32/1 -> Detect Increase3/1
  Detect Increase2/1 -> SR_Latch20/1
  Relational Operator6/1 -> AND1/1
  Abs10/1 -> Relational Operator6/1
  [VTQD_RFWhlQuickSkip_flg] -> AND14/1
  Constant12/1 -> Delay8/2
  [VTQR_NoABSREDUWhlTqReq_Nm] -> Delay11/1
  Relational Operator71/1 -> AND31/1
  [VTQD_BrkSwSta_flg] -> OR11/3
  Constant71/1 -> Delay1/2
  Delay3/1 -> Add/2
  Constant3/1 -> Relational Operator2/2
  [VTQR_NoABSFEDUWhlTqReq_Nm] -> Delay12/1
  [VTQD_RRWhlQuickSkip_flg] -> AND53/3
  Add40/1 -> Relational Operator64/1
  [VINP_FrPTCSActive_flg] -> OR11/1
  [VINP_RRRawWhlSpeed_kph] -> Add21/2
  OR23/1 -> SR_Latch15/2
  Detect Decrease/1 -> SR_Latch7/1
  SR_Latch11/1 -> OR18/1  "VTQD_PosFrontWhlSkip_flg"
  Constant43/1 -> Relational Operator37/2
  Constant55/1 -> Relational Operator61/2
  [VTQD_LFRRWhlSkip_flg] -> AND41/1
  [VTQD_LRWhlQuickSkip_flg] -> AND50/3
  Relational Operator41/1 -> AND15/4
  Detect Increase6/1 -> SR_Latch25/1
  AND28/1 -> OR24/2
  [VINP_RRRawWhlSpeed_kph] -> Add17/1
  [VTQD_RFLRWhlSkip_flg] -> OR22/6
  [VINP_RRRawWhlSpeed_kph] -> Delay6/1
  [VINP_RFRawWhlSpeed_kph] -> Relational Operator65/2
  Constant24/1 -> Relational Operator23/2
  OR15/1 -> [VTQD_RightWhlSkip_flg]  "VTQD_RightWhlSkip_flg"
  [VINP_LRRawWhlSpeed_kph] -> Add6/1
  OR33/1 -> Detect Increase4/1
  Abs34/1 -> Relational Operator60/1
  SR_Latch24/1 -> [VTQD_TripleWhlSkip_flg]  "VTQD_TripleWhlSkip_flg"
  [VTQD_RRWhlQuickSkip_flg] -> NOT3/1
  [VINP_RRRawWhlSpeed_kph] -> Add31/2
  [VINP_LRRawWhlSpeed_kph] -> Add14/1
  [VTQD_LRWhlQuickSkip_flg] -> AND10/2
  OR29/1 -> [VTQD_RFLRWhlSkip_flg]  "VTQD_RFLRWhlSkip_flg"
  Relational Operator30/1 -> AND6/4
  [VTQR_NoABSFEDUWhlTqReq_Nm] -> Delay34/1
  Constant6/1 -> Relational Operator5/2
  AND35/1 -> OR31/2
  SR_Latch6/1 -> OR9/2  "VTQD_NegLeftWhlSkip_flg"
  [VTQD_LFWhlQuickSkip_flg] -> AND54/2
  [VINP_LRRawWhlSpeed_kph] -> Relational Operator66/2
  Constant61/1 -> Relational Operator73/2
  AND7/1 -> OR7/1
  OR36/1 -> SR_Latch24/2
  [VTQR_NoABSREDUWhlTqReq_Nm] -> Delay33/1
  [VINP_LFRawWhlSpeed_kph] -> Relational Operator32/1
  Relational Operator22/1 -> AND4/2
  Relational Operator14/1 -> AND3/1
  Delay1/1 -> Add4/2
  Relational Operator32/1 -> AND7/1
  [VINP_RFRawWhlSpeed_kph] -> Add12/1
  Abs20/1 -> Relational Operator21/1
  Delay19/1 -> Add32/2
  AND25/1 -> [VTQD_DiagonalWhlSkip_flg]  "VTQD_DiagonalWhlSkip_flg"
  Abs17/1 -> Relational Operator14/1
  [VTQD_LFWhlQuickSkip_flg] -> AND42/1
  [VINP_VehSpeed_kph] -> Delay8/1
  Relational Operator46/1 -> AND16/3
  [VTQD_LFWhlQuickSkip_flg] -> AND10/1
  Relational Operator37/1 -> AND11/2
  Relational Operator67/1 -> AND29/4
  Relational Operator42/1 -> AND15/1
  Abs35/1 -> Relational Operator61/1
  Delay33/1 -> Add44/2
  [VTQD_DoubleWhlSkip_flg] -> OR6/1
  [VTQD_LFWhlQuickSkip_flg] -> AND37/2
  [VTQD_RearLFWhlSkip_flg] -> AND59/1
  [VTQD_FrontRearWhlSkip_flg] -> AND18/3
  [VINP_RRRawWhlSpeed_kph] -> Relational Operator53/2
  AND12/1 -> OR14/2
  Delay22/1 -> Add35/2
  AND10/1 -> OR8/2
  [VTQD_RearRFWhlSkip_flg] -> OR35/4
  [VTQR_NoABSFEDUWhlTqReq_Nm] -> Delay20/1
  [VTQR_NoABSREDUWhlTqReq_Nm] -> Delay27/1
  [VINP_LRRawWhlSpeed_kph] -> Add23/1
  [VINP_LRRawWhlSpeed_kph] -> Add16/1
  [VINP_LFRawWhlSpeed_kph] -> Relational Operator52/1
  Delay26/1 -> Add41/2
  [VTQD_LFWhlQuickSkip_flg] -> AND60/2
  Constant18/1 -> Relational Operator12/2
  AND24/1 -> OR20/1
  [VTQD_RightWhlSkip_flg] -> AND40/1
  Constant25/1 -> Relational Operator21/2
  SR_Latch19/1 -> OR29/2  "VTQD_NegRFLRWhlSkip_flg"
  Delay23/1 -> Add34/2
  OR35/1 -> SR_Latch24/1
  [VTQD_GearActualPosn_enum] -> Equal1/1
  SR_Latch10/1 -> OR15/2  "VTQD_NegRightWhlSkip_flg"
  Relational Operator56/1 -> AND22/2
  OR30/1 -> [VTQD_AllWhlStable_flg]  "VTQD_AllWhlStable_flg"
  SR_Latch8/1 -> OR12/3
  [VINP_LFRawWhlSpeed_kph] -> Add15/2
  Whleels State Machine/1(VTQD_WhlSkipSta_enum) -> Switch2/3
  Add31/1 -> Abs33/1
  [VTQD_AllWhlSkip_flg] -> OR36/1
  Constant63/1 -> Equal1/2
  Bus Selector1/2 -> [VTQD_VehActSpd_kph]  "<VTQD_VehActSpd_kph>"
  BMain_outputs/1 -> Bus Selector2/1
  Bus Selector2/1 -> [VTQR_NoABSFEDUWhlTqReq_Nm]  "<VTQR_NoABSFEDUWhlTqReq_Nm>"
  Bus Selector2/2 -> [VTQR_NoABSREDUWhlTqReq_Nm]  "<VTQR_NoABSREDUWhlTqReq_Nm>"
  Bus Selector/10 -> [VINP_DIDGetDynoMode_flg]  "<VINP_DIDGetDynoMode_flg>"
  [VINP_DIDGetDynoMode_flg] -> Whleels State Machine/19(VINP_DIDGetDynoMode_flg)

== system tqdtqr_rebuild_V3/Input_Convert/Signal function/combo key ==
  BSCPIn_outputs : Inport
  BSignalConvert_outputs : Inport  Port=2
  Bus Selector : BusSelector  OutputSignals=task_time_s,VINP_SWCRegenUp_flg,VINP_SWCRegenDown_flg,VINP_SWC2LScrollUpSta_flg,VINP_SWC2LScrollDownSta_flg,VINP_SWC2RScrollUpSta_flg,VINP_SWC2RScrollDownSta_flg,VINP_SWC2LScrollPressSta_flg,VINP_SWC2RScrollPressSta_flg,VINP_SWC2LADASSta_flg,VINP_SWC2LDriveModeSta_flg,VINP_SWC2RRightSta_flg,VINP_SWC2RLeftSta_flg,VPMM_PowerSta_enum
  Bus Selector1 : BusSelector  OutputSignals=VTQD_ShiftGearPosn_enum
  Combo Key Detection : Subsystem
  Mode Coordination : Subsystem
  Operation Condition : Subsystem
  Signal Status Detection : Subsystem
  VTQD_ComboKeyPreEn_flg : Outport
  VTQD_ComboKeyEn_flg : Outport  Port=2
  VTQD_SysMode_enum : Outport  Port=3
  wires:
  BSCPIn_outputs/1 -> Bus Selector/1
  Bus Selector/1 -> [task_time_s]  "<task_time_s>"
  Bus Selector/2 -> [VINP_SWCRegenUp_flg]  "<VINP_SWCRegenUp_flg>"
  Bus Selector/3 -> [VINP_SWCRegenDown_flg]  "<VINP_SWCRegenDown_flg>"
  Bus Selector/4 -> [VINP_SWCResUpSta_flg]  "<VINP_SWC2LScrollUpSta_flg>"
  Bus Selector/5 -> [VINP_SWCSetdownSta_flg]  "<VINP_SWC2LScrollDownSta_flg>"
  Bus Selector/6 -> [VINP_SWCUpSta_flg]  "<VINP_SWC2RScrollUpSta_flg>"
  Bus Selector/7 -> [VINP_SWCDownSta_flg]  "<VINP_SWC2RScrollDownSta_flg>"
  Bus Selector/8 -> [VINP_SWCCANCELSta_flg]  "<VINP_SWC2LScrollPressSta_flg>"
  Bus Selector/9 -> [VINP_SWCmodeSta_flg]  "<VINP_SWC2RScrollPressSta_flg>"
  Bus Selector/10 -> [VINP_SWCACCSta_flg]  "<VINP_SWC2LADASSta_flg>"
  Bus Selector/11 -> [VINP_SWCDistanceSta_flg]  "<VINP_SWC2LDriveModeSta_flg>"
  Bus Selector/12 -> [VINP_SWCRightSta_flg]  "<VINP_SWC2RRightSta_flg>"
  Bus Selector/13 -> [VINP_SWCLeftSta_flg]  "<VINP_SWC2RLeftSta_flg>"
  Bus Selector/14 -> [VPMM_PowerSta_enum]  "<VPMM_PowerSta_enum>"
  BSignalConvert_outputs/1 -> Bus Selector1/1
  Bus Selector1/1 -> [VTQD_ShiftGearPosn_enum]  "<VTQD_ShiftGearPosn_enum>"
  [VTQD_ComboKeyPreEn_flg] -> VTQD_ComboKeyPreEn_flg/1
  [VTQD_ComboKeyEn_flg] -> VTQD_ComboKeyEn_flg/1
  [VTQD_SysMode_enum] -> VTQD_SysMode_enum/1
  Signal Status Detection/3(VSCP_ComboKeyReset_flg) -> [VSCP_ComboKeyReset_flg]
  [VINP_SWCCANCELSta_flg] -> Signal Status Detection/8(VINP_SWCCANCELSta_flg)
  Signal Status Detection/2(VSCP_ComboKeyEnCMD_flg) -> [VSCP_ComboKeyEnCMD_flg]
  [VPMM_PowerSta_enum] -> Operation Condition/1(VINP_PwrSta_enum)
  [VINP_SWCResUpSta_flg] -> Signal Status Detection/4(VINP_SWCResUpSta_flg)
  [VINP_SWCSetdownSta_flg] -> Signal Status Detection/5(VINP_SWCSetdownSta_flg)
  [VINP_SWCUpSta_flg] -> Signal Status Detection/6(VINP_SWCUpSta_flg)
  Signal Status Detection/1(VSCP_ComboKey_enum) -> [VSCP_ComboKey_enum]
  [VTQD_ComboKeyPreEn_flg] -> Signal Status Detection/9(VSCP_ComboKeyPreEn_flg)
  [VTQD_ComboKeyEn_flg] -> Signal Status Detection/16(VSCP_ComboKeyEn_flg)
  [VSCP_ComboKey_enum] -> Combo Key Detection/4(VSCP_ComboKey_enum)
  [task_time_s] -> Combo Key Detection/1(TASK_TIME_10_MS)
  [VTQD_ComboKeyEn_flg] -> Combo Key Detection/2(VSCP_ComboKeyEn_flg)
  [task_time_s] -> Signal Status Detection/1(TASK_TIME_10_MS)
  [VSCP_ComboKeyReset_flg] -> Combo Key Detection/3(VSCP_ComboKeyReset_flg)
  Signal Status Detection/5(VSCP_StreetFightModeOff_flg) -> [VSCP_StreetFightModeOff_flg]
  [VINP_SWCDistanceSta_flg] -> Signal Status Detection/12(VINP_SWCDistanceSta_flg)
  [VTQD_SysMode_enum] -> Signal Status Detection/11(VSCP_SysMode_enum)
  Signal Status Detection/4(VSCP_ComboKeyEnter_flg) -> [VSCP_ComboKeyEnter_flg]
  [VINP_SWCRegenUp_flg] -> Signal Status Detection/3(VINP_SWCRegenUp_flg)
  [VINP_SWCRightSta_flg] -> Signal Status Detection/14(VINP_SWCRightSta_flg)
  [VINP_SWCACCSta_flg] -> Signal Status Detection/10(VINP_SWCACCSta_flg)
  [VSCP_ManufactureMode_flg] -> Mode Coordination/3(VSCP_ManufactureMode_flg)
  [VSCP_ExhibitionMode_flg] -> Mode Coordination/4(VSCP_ExhibitionMode_flg)
  Mode Coordination/1(VSCP_SysMode_enum) -> [VTQD_SysMode_enum]
  [VTQD_ShiftGearPosn_enum] -> Operation Condition/2(VINP_ShiftGearPosn_enum)
  Operation Condition/1(VSCP_ComboKeyPreEn_flg) -> [VTQD_ComboKeyPreEn_flg]
  Combo Key Detection/4(VSCP_ExhibitionMode_flg) -> [VSCP_ExhibitionMode_flg]
  [VSCP_DiagnosisOffMode_flg] -> Mode Coordination/5(VSCP_DiagnosisOffMode_flg)
  [VSCP_StreetFightModeOff_flg] -> Combo Key Detection/6(VSCP_StreetFightModeOff_flg)
  [VSCP_ComboKeyEnter_flg] -> Combo Key Detection/5(VSCP_ComboKeyEnter_flg)
  Operation Condition/2(VSCP_ComboKeyEn_flg) -> [VTQD_ComboKeyEn_flg]
  [VINP_SWCLeftSta_flg] -> Signal Status Detection/15(VINP_SWCLeftSta_flg)
  Combo Key Detection/1(VSCP_StreetFightMode_flg) -> [VSCP_StreetFightMode_flg]
  [VINP_SWCmodeSta_flg] -> Signal Status Detection/13(VINP_SWCmodeSta_flg)
  [VSCP_EngineeringMode_flg] -> Mode Coordination/2(VSCP_EngineeringMode_flg)
  [VINP_SWCRegenDown_flg] -> Signal Status Detection/2(VINP_SWCRegenDown_flg)
  [VSCP_StreetFightMode_flg] -> Mode Coordination/1(VSCP_StreetFightMode_flg)
  Combo Key Detection/3(VSCP_ManufactureMode_flg) -> [VSCP_ManufactureMode_flg]
  Combo Key Detection/5(VSCP_DiagnosisOffMode_flg) -> [VSCP_DiagnosisOffMode_flg]
  Combo Key Detection/2(VSCP_EngineeringMode_flg) -> [VSCP_EngineeringMode_flg]
  [VSCP_ComboKeyEnCMD_flg] -> Operation Condition/3(VSCP_ComboKeyEnCMD_flg)
  [VINP_SWCDownSta_flg] -> Signal Status Detection/7(VINP_SWCDownSta_flg)

== system tqdtqr_rebuild_V3/SCP_In/Input Signal/BrkPedalPos ==
  Inp_signal : Inport
  Invalid_condition : Inport  Port=2
  Constant24 : Constant  Value=FALSE
  Switch : Switch  Criteria=u2 ~= 0
      settings: AttributesFormatString=%<Criteria>
  Out_signal : Outport
  wires:
  Switch/1 -> Out_signal/1
  Invalid_condition/1 -> Switch/2
  Inp_signal/1 -> Switch/1
  Constant24/1 -> Switch/3

== system tqdtqr_rebuild_V3/SCP_In/Input Signal/BrkSwSta ==
  Inp_signal : Inport
  Invalid_condition : Inport  Port=2
  Constant24 : Constant  Value=FALSE
  Switch : Switch  Criteria=u2 ~= 0
      settings: AttributesFormatString=%<Criteria>
  Out_signal : Outport
  wires:
  Invalid_condition/1 -> Switch/2
  Switch/1 -> Out_signal/1
  Inp_signal/1 -> Switch/1
  Constant24/1 -> Switch/3

== system tqdtqr_rebuild_V3/SCP_In/Input Signal/ShifterFailsta ==
  Inp_signal : Inport
  Invalid_condition : Inport  Port=2
  Constant24 : Constant  Value=ENUM_SHIFTERERRSTA_SHIFTERFAILURE
  Switch : Switch  Criteria=u2 ~= 0
      settings: AttributesFormatString=%<Criteria>
  Out_signal : Outport
  wires:
  Constant24/1 -> Switch/1
  Switch/1 -> Out_signal/1
  Invalid_condition/1 -> Switch/2
  Inp_signal/1 -> Switch/3

== system tqdtqr_rebuild_V3/SCP_In/Input Signal/ShifterHandleCmd ==
  Inp_signal : Inport
  Invalid_condition : Inport  Port=2
  Constant24 : Constant  Value=KTQD_VirtualShifterCMD_enum
  Switch : Switch  Criteria=u2 ~= 0
      settings: AttributesFormatString=%<Criteria>
  Out_signal : Outport
  wires:
  Inp_signal/1 -> Switch/3
  Invalid_condition/1 -> Switch/2
  Switch/1 -> Out_signal/1
  Constant24/1 -> Switch/1

== system tqdtqr_rebuild_V3/SCP_In/Input Signal/VDDM_LimpHomeAct_flg_ovrd ==
  Signal_In : Inport
  Constant1 : Constant  Value=KTQD_LimpHomeAct_flg_ovrdval
  Constant2 : Constant  Value=KTQD_LimpHomeAct_flg_ovrdflg
  Switch : Switch  Criteria=u2 ~= 0
      settings: AttributesFormatString=%<Criteria>
  Signal_Out : Outport
  wires:
  Signal_In/1 -> Switch/3
  Switch/1 -> Signal_Out/1
  Constant2/1 -> Switch/2
  Constant1/1 -> Switch/1

== system tqdtqr_rebuild_V3/SCP_In/Input Signal/VDHP_LowIdleAccPedal_flg_ovrd ==
  Signal_In : Inport
  Constant42 : Constant  Value=KTQD_LowIdle_flg_ovrdflg  OutDataTypeStr=Inherit: Inherit via back propagation
  Constant43 : Constant  Value=KTQD_LowIdle_flg_ovrdval  OutDataTypeStr=Inherit: Inherit via back propagation
  LiuzgSwitch15 : Switch  Criteria=u2 ~= 0
      settings: AttributesFormatString=<%<Criteria>>
  Signal_Out : Outport
  wires:
  Constant42/1 -> LiuzgSwitch15/2
  Constant43/1 -> LiuzgSwitch15/1
  LiuzgSwitch15/1 -> Signal_Out/1
  Signal_In/1 -> LiuzgSwitch15/3
